simulink subsystem "proc_nav_ros_input"  (R2024b)
settings: Solver=VariableStepAuto  StartTime=0.0  StopTime=10.0  RelTol=1e-3
undefined symbols (not defined in the file or in its folder): simulink
libraries: ros2lib x9, simulink x2
settings Model: Creator=relat  LastModifiedBy=nimai

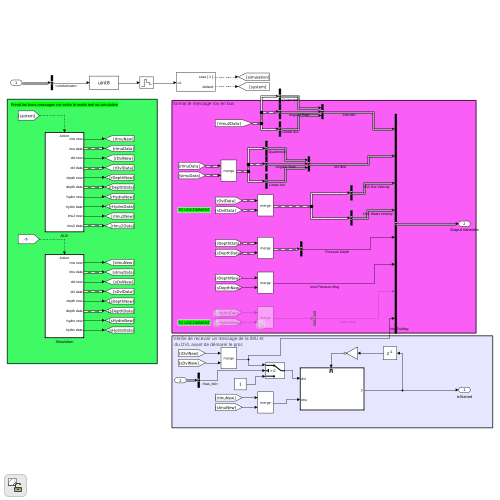
[thumbnail: Simulink's stored preview of the top-level diagram]
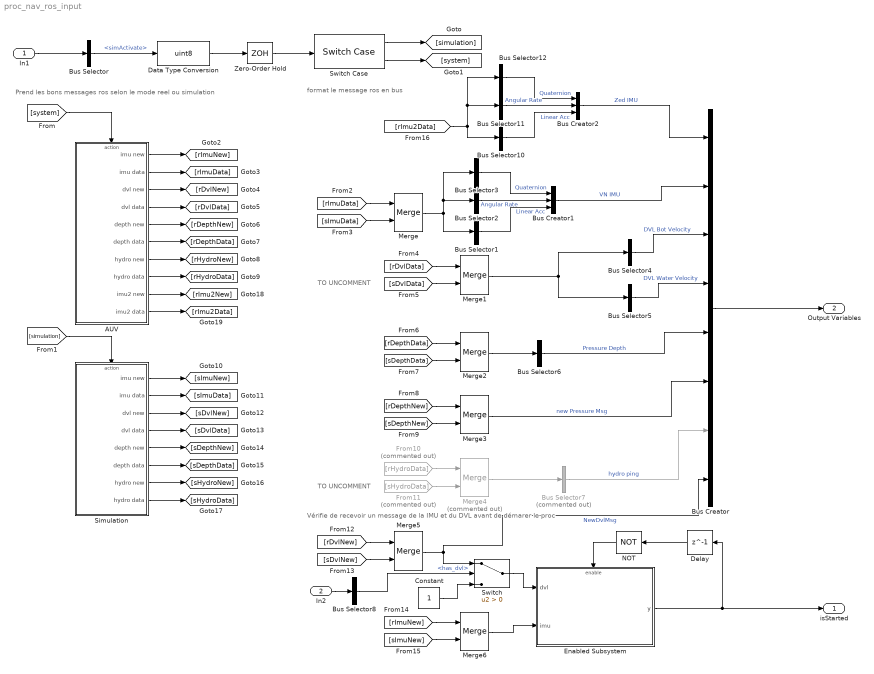
== system proc_nav_ros_input ==
  note: Vérifie de recevoir un message de la IMU et
      |  du DVL avant de démarer le proc
  note: format le message ros en bus
  note: TO UNCOMMENT
  note: Prend les bons messages ros selon le mode reel ou simulation
  note: TO UNCOMMENT
  In1 : Inport
  In2 : Inport  Port=2
  AUV : Subsystem  TreatAsAtomicUnit=on
  Bus Creator : BusCreator  Inputs=8
  Bus Creator1 : BusCreator  Inputs=3
  Bus Creator2 : BusCreator  Inputs=3
  Bus Selector : BusSelector  OutputSignals=simActivate
  Bus Selector1 : BusSelector  OutputSignals=linear_acceleration  OutputAsBus=on
  Bus Selector10 : BusSelector  OutputSignals=linear_acceleration  OutputAsBus=on
  Bus Selector11 : BusSelector  OutputSignals=angular_velocity  OutputAsBus=on
  Bus Selector12 : BusSelector  OutputSignals=orientation  OutputAsBus=on
  Bus Selector2 : BusSelector  OutputSignals=angular_velocity  OutputAsBus=on
  Bus Selector3 : BusSelector  OutputSignals=orientation  OutputAsBus=on
  Bus Selector4 : BusSelector  OutputSignals=x_vel_btm,y_vel_btm,z_vel_btm,e_vel_btm  OutputAsBus=on
  Bus Selector5 : BusSelector  OutputSignals=velocity1,velocity2,velocity3,velocity4  OutputAsBus=on
  Bus Selector6 : BusSelector  OutputSignals=data  OutputAsBus=on
  Bus Selector7 : BusSelector  Commented=on  OutputSignals=heading,elevation  OutputAsBus=on
  Bus Selector8 : BusSelector  OutputSignals=has_dvl
  Constant : Constant
  Data Type Conversion : DataTypeConversion  OutDataTypeStr=uint8  SaturateOnIntegerOverflow=off  RndMeth=Floor
  Delay : Delay  DelayLength=1  InitialCondition=0
  Enabled Subsystem : Subsystem  TreatAsAtomicUnit=on
  From10 : From  Commented=on  GotoTag=rHydroData
  From11 : From  Commented=on  GotoTag=sHydroData
  Merge{,1..3,5..6} (6 alike) : Merge
  Merge4 : Merge  Commented=on
  NOT : Logic  Operator=NOT  IconShape=distinctive  AllPortsSameDT=off  OutDataTypeStr=boolean
  Simulation : Subsystem  TreatAsAtomicUnit=on
  Switch : Switch  Criteria=u2 > Threshold  SaturateOnIntegerOverflow=off  InputSameDT=off
  Switch Case : SwitchCase
  Zero-Order Hold : ZeroOrderHold  SampleTime=simulink.procNav.sampletime
  isStarted : Outport
  Output Variables : Outport  Port=2
  wires:
  In1/1 -> Bus Selector/1
  Bus Selector/1 -> Data Type Conversion/1  "<simActivate>"
  Data Type Conversion/1 -> Zero-Order Hold/1
  Zero-Order Hold/1 -> Switch Case/1
  Switch Case/1 -> [simulation]
  Switch Case/2 -> [system]
  [system] -> AUV/Action
  AUV/1(imu new) -> [rImuNew]
  AUV/2(imu data) -> [rImuData]
  AUV/3(dvl new) -> [rDvlNew]
  AUV/4(dvl data) -> [rDvlData]
  AUV/5(depth new) -> [rDepthNew]
  AUV/6(depth data) -> [rDepthData]
  AUV/7(hydro new) -> [rHydroNew]
  AUV/8(hydro data) -> [rHydroData]
  Simulation/5(depth new) -> [sDepthNew]
  Simulation/4(dvl data) -> [sDvlData]
  Simulation/7(hydro new) -> [sHydroNew]
  Simulation/2(imu data) -> [sImuData]
  Simulation/1(imu new) -> [sImuNew]
  [simulation] -> Simulation/Action
  Simulation/6(depth data) -> [sDepthData]
  Simulation/3(dvl new) -> [sDvlNew]
  Simulation/8(hydro data) -> [sHydroData]
  [rImuData] -> Merge/1
  [sImuData] -> Merge/2
  Merge/1 -> Bus Selector2/1, Bus Selector3/1, Bus Selector1/1
  [rDvlData] -> Merge1/1
  [sDvlData] -> Merge1/2
  [sDepthData] -> Merge2/2
  [rDepthData] -> Merge2/1
  Merge2/1 -> Bus Selector6/1
  [rDepthNew] -> Merge3/1
  [sDepthNew] -> Merge3/2
  From10/1 -> Merge4/1
  From11/1 -> Merge4/2
  Merge4/1 -> Bus Selector7/1
  Bus Selector3/1 -> Bus Creator1/1  "Quaternion"
  Bus Selector2/1 -> Bus Creator1/2  "Angular Rate"
  Bus Selector1/1 -> Bus Creator1/3  "Linear Acc"
  Bus Selector4/1 -> Bus Creator/3  "DVL Bot Velocity"
  Bus Selector5/1 -> Bus Creator/4  "DVL Water Velocity"
  Bus Selector6/1 -> Bus Creator/5  "Pressure Depth"
  Merge3/1 -> Bus Creator/6  "new Pressure Msg"
  Bus Selector7/1 -> Bus Creator/7  "hydro ping"
  [sDvlNew] -> Merge5/2
  [rDvlNew] -> Merge5/1
  [sImuNew] -> Merge6/2
  [rImuNew] -> Merge6/1
  Merge5/1 -> Bus Creator/8, Switch/1  "NewDvlMsg"
  Merge6/1 -> Enabled Subsystem/2(imu)
  Enabled Subsystem/1(y) -> isStarted/1, Delay/1
  Delay/1 -> NOT/1
  NOT/1 -> Enabled Subsystem/Enable
  Bus Creator/1 -> Output Variables/1
  Merge1/1 -> Bus Selector5/1, Bus Selector4/1
  In2/1 -> Bus Selector8/1
  Bus Selector8/1 -> Switch/2  "<has_dvl>"
  Switch/1 -> Enabled Subsystem/1(dvl)
  Constant/1 -> Switch/3
  AUV/9(imu2 new) -> [rImu2New]
  AUV/10(imu2 data) -> [rImu2Data]
  Bus Creator1/1 -> Bus Creator/2  "VN IMU"
  [rImu2Data] -> Bus Selector10/1, Bus Selector11/1, Bus Selector12/1
  Bus Selector10/1 -> Bus Creator2/3  "Linear Acc"
  Bus Creator2/1 -> Bus Creator/1  "Zed IMU"
  Bus Selector11/1 -> Bus Creator2/2  "Angular Rate"
  Bus Selector12/1 -> Bus Creator2/1  "Quaternion"

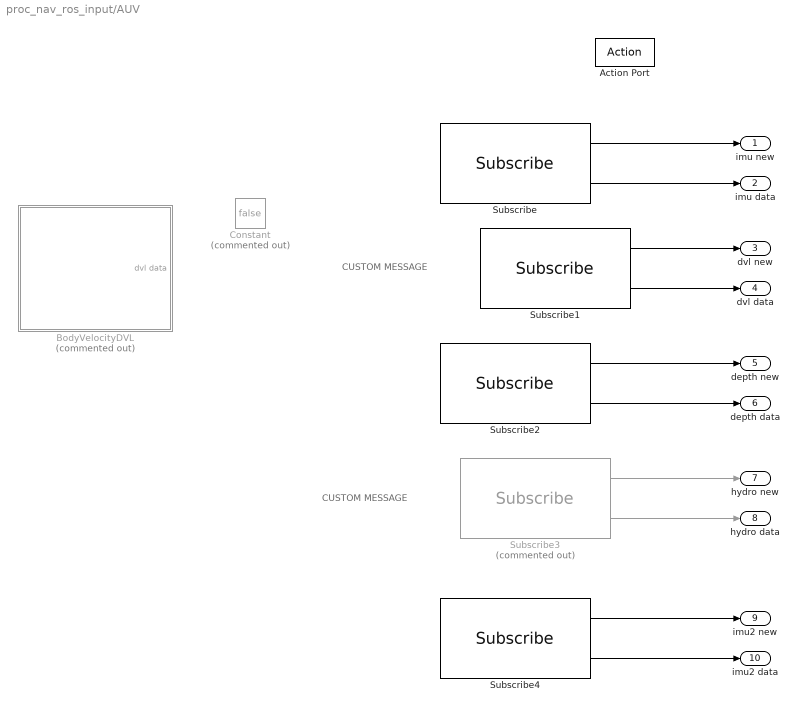
== system proc_nav_ros_input/AUV ==
  note: CUSTOM MESSAGE
  note: CUSTOM MESSAGE
  Action Port : ActionPort
  BodyVelocityDVL : Subsystem  Commented=on
  Constant : Constant  Commented=on  Value=false  VectorParams1D=off  SampleTime=-1
  Subscribe : ros2lib/Subscribe  topicSource=Specify your own  topic=/provider_imu/imu_info  messageType=sensor_msgs/Imu  sampleTime=simulink.procNav.sampletime  QOSHistory=Keep last  QOSDepth=10  QOSReliability=Reliable  QOSDurability=Volatile  QOSDeadline=inf  QOSLifespan=inf  QOSLiveliness=Automatic  QOSLeaseDuration=inf  QOSAvoidROSNamespaceConventions=off
  Subscribe1 : ros2lib/Subscribe  topicSource=Specify your own  topic=/provider_dvl/dvl_velocity  messageType=sonia_common_ros2/BodyVelocityDVL  sampleTime=simulink.procNav.sampletime  QOSHistory=Keep last  QOSDepth=10  QOSReliability=Reliable  QOSDurability=Volatile  QOSDeadline=inf  QOSLifespan=inf  QOSLiveliness=Automatic  QOSLeaseDuration=inf  QOSAvoidROSNamespaceConventions=off
  Subscribe2 : ros2lib/Subscribe  topicSource=Specify your own  topic=/provider_depth/depth  messageType=std_msgs/Float32  sampleTime=simulink.procNav.sampletime  QOSHistory=Keep last  QOSDepth=10  QOSReliability=Reliable  QOSDurability=Volatile  QOSDeadline=inf  QOSLifespan=inf  QOSLiveliness=Automatic  QOSLeaseDuration=inf  QOSAvoidROSNamespaceConventions=off
  Subscribe3 : ros2lib/Subscribe  Commented=on  topicSource=Specify your own  topic=/proc_hydro/ping  messageType=sonia_common_ros2/PingAngles  sampleTime=simulink.procNav.sampletime  QOSHistory=Keep last  QOSDepth=1  QOSReliability=Reliable  QOSDurability=Volatile  QOSDeadline=5  QOSLifespan=5  QOSLiveliness=Automatic  QOSLeaseDuration=5  QOSAvoidROSNamespaceConventions=off
  Subscribe4 : ros2lib/Subscribe  topicSource=Specify your own  topic=/zed/zed_node/imu/data  messageType=sensor_msgs/Imu  sampleTime=simulink.procNav.sampletime  QOSHistory=Keep last  QOSDepth=10  QOSReliability=Reliable  QOSDurability=Volatile  QOSDeadline=Inf  QOSLifespan=Inf  QOSLiveliness=Automatic  QOSLeaseDuration=Inf  QOSAvoidROSNamespaceConventions=off
  imu new : Outport
  imu data : Outport  Port=2
  dvl new : Outport  Port=3
  dvl data : Outport  Port=4
  depth new : Outport  Port=5
  depth data : Outport  Port=6
  hydro new : Outport  Port=7
  hydro data : Outport  Port=8
  imu2 new : Outport  Port=9
  imu2 data : Outport  Port=10
  wires:
  Subscribe4/2 -> imu2 data/1
  Subscribe4/1 -> imu2 new/1
  Subscribe1/2 -> dvl data/1
  Subscribe2/2 -> depth data/1
  Subscribe2/1 -> depth new/1
  Subscribe1/1 -> dvl new/1
  Subscribe/2 -> imu data/1
  Subscribe/1 -> imu new/1
  Subscribe3/1 -> hydro new/1
  Subscribe3/2 -> hydro data/1

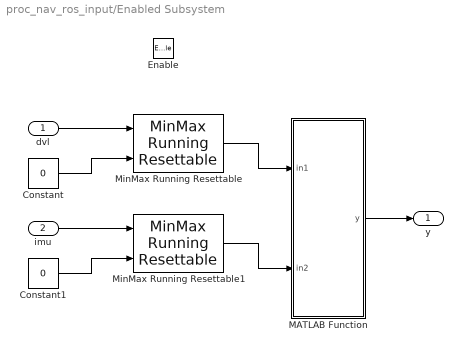
== system proc_nav_ros_input/Enabled Subsystem ==
  dvl : Inport
  imu : Inport  Port=2
  Enable : EnablePort
  Constant : Constant  Value=0
  Constant1 : Constant  Value=0
  MATLAB Function : MATLAB Function  TreatAsAtomicUnit=on
  MinMax Running Resettable : simulink/Math Operations/MinMax Running Resettable  Function=max  vinit=0.0
  MinMax Running Resettable1 : simulink/Math Operations/MinMax Running Resettable  Function=max  vinit=0.0
  y : Outport
  wires:
  MATLAB Function/1(y) -> y/1
  MinMax Running Resettable1/1 -> MATLAB Function/2(in2)
  MinMax Running Resettable/1 -> MATLAB Function/1(in1)
  imu/1 -> MinMax Running Resettable1/1
  Constant1/1 -> MinMax Running Resettable1/2
  Constant/1 -> MinMax Running Resettable/2
  dvl/1 -> MinMax Running Resettable/1

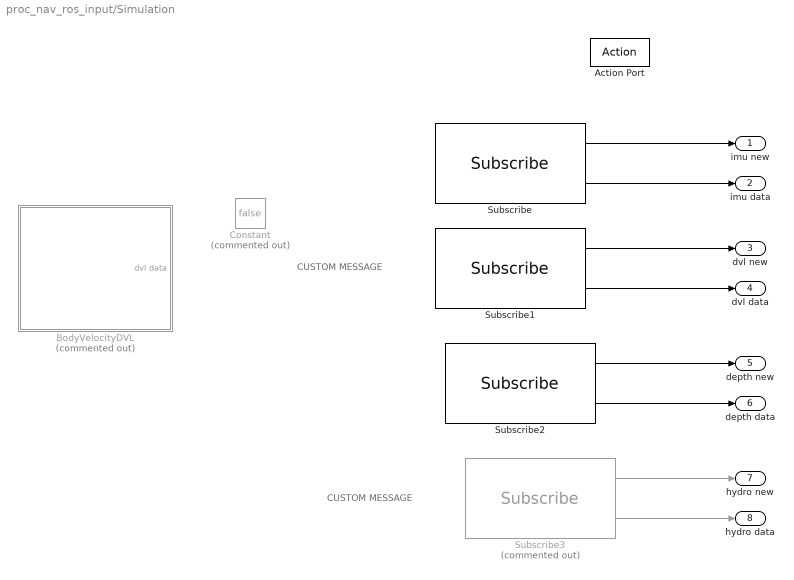
== system proc_nav_ros_input/Simulation ==
  note: CUSTOM MESSAGE
  note: CUSTOM MESSAGE
  Action Port : ActionPort
  BodyVelocityDVL : Subsystem  Commented=on
  Constant : Constant  Commented=on  Value=false  VectorParams1D=off
  Subscribe : ros2lib/Subscribe  topicSource=Specify your own  topic=/proc_simulation/imu_info  messageType=sensor_msgs/Imu  sampleTime=simulink.procNav.sampletime  QOSHistory=Keep last  QOSDepth=10  QOSReliability=Reliable  QOSDurability=Volatile  QOSDeadline=inf  QOSLifespan=inf  QOSLiveliness=Automatic  QOSLeaseDuration=inf  QOSAvoidROSNamespaceConventions=off
  Subscribe1 : ros2lib/Subscribe  topicSource=Specify your own  topic=/proc_simulation/dvl_velocity  messageType=sonia_common_ros2/BodyVelocityDVL  sampleTime=simulink.procNav.sampletime  QOSHistory=Keep last  QOSDepth=10  QOSReliability=Reliable  QOSDurability=Volatile  QOSDeadline=inf  QOSLifespan=inf  QOSLiveliness=Automatic  QOSLeaseDuration=inf  QOSAvoidROSNamespaceConventions=off
  Subscribe2 : ros2lib/Subscribe  topicSource=Specify your own  topic=/proc_simulation/depth  messageType=std_msgs/Float32  sampleTime=simulink.procNav.sampletime  QOSHistory=Keep last  QOSDepth=10  QOSReliability=Reliable  QOSDurability=Volatile  QOSDeadline=inf  QOSLifespan=inf  QOSLiveliness=Automatic  QOSLeaseDuration=inf  QOSAvoidROSNamespaceConventions=off
  Subscribe3 : ros2lib/Subscribe  Commented=on  topicSource=Specify your own  topic=/proc_simulation/ping  messageType=sonia_common_ros2/PingAngles  sampleTime=simulink.procNav.sampletime  QOSHistory=Keep last  QOSDepth=1  QOSReliability=Reliable  QOSDurability=Volatile  QOSDeadline=5  QOSLifespan=5  QOSLiveliness=Automatic  QOSLeaseDuration=5  QOSAvoidROSNamespaceConventions=off
  imu new : Outport
  imu data : Outport  Port=2
  dvl new : Outport  Port=3
  dvl data : Outport  Port=4
  depth new : Outport  Port=5
  depth data : Outport  Port=6
  hydro new : Outport  Port=7
  hydro data : Outport  Port=8
  wires:
  Subscribe1/2 -> dvl data/1
  Subscribe2/2 -> depth data/1
  Subscribe2/1 -> depth new/1
  Subscribe1/1 -> dvl new/1
  Subscribe/2 -> imu data/1
  Subscribe/1 -> imu new/1
  Subscribe3/1 -> hydro new/1
  Subscribe3/2 -> hydro data/1

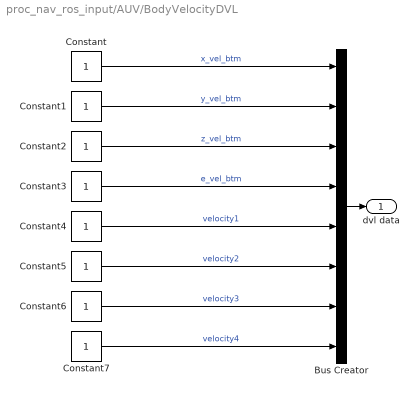
== system proc_nav_ros_input/AUV/BodyVelocityDVL ==
  Bus Creator : BusCreator  Inputs=8
  Constant{,1..7} (8 alike) : Constant  SampleTime=-1
  dvl data : Outport
  wires:
  Constant/1 -> Bus Creator/1  "x_vel_btm"
  Constant4/1 -> Bus Creator/5  "velocity1"
  Constant6/1 -> Bus Creator/7  "velocity3"
  Constant3/1 -> Bus Creator/4  "e_vel_btm"
  Constant5/1 -> Bus Creator/6  "velocity2"
  Bus Creator/1 -> dvl data/1
  Constant7/1 -> Bus Creator/8  "velocity4"
  Constant1/1 -> Bus Creator/2  "y_vel_btm"
  Constant2/1 -> Bus Creator/3  "z_vel_btm"

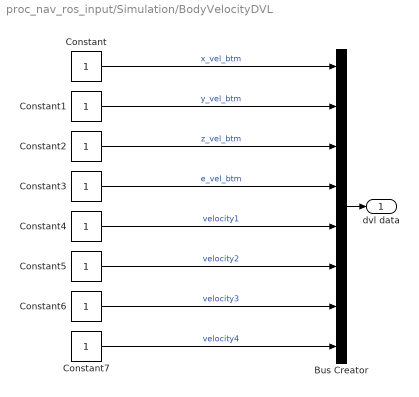
== system proc_nav_ros_input/Simulation/BodyVelocityDVL ==
  Bus Creator : BusCreator  Inputs=8
  Constant{,1..7} (8 alike) : Constant
  dvl data : Outport
  wires:
  Constant/1 -> Bus Creator/1  "x_vel_btm"
  Constant4/1 -> Bus Creator/5  "velocity1"
  Constant6/1 -> Bus Creator/7  "velocity3"
  Constant3/1 -> Bus Creator/4  "e_vel_btm"
  Constant5/1 -> Bus Creator/6  "velocity2"
  Bus Creator/1 -> dvl data/1
  Constant7/1 -> Bus Creator/8  "velocity4"
  Constant1/1 -> Bus Creator/2  "y_vel_btm"
  Constant2/1 -> Bus Creator/3  "z_vel_btm"

== matlab function proc_nav_ros_input/Enabled Subsystem/MATLAB Function ==
  data: in1 input; y output; in2 input
function y = fcn(in1,in2)
    if in1+in2 >=2
        y=1;
    else
        y=0;
    end
end
